simulink model "Problem1"  (R2020b)
settings: Solver=VariableStepAuto  StartTime=0.0  StopTime=10  RelTol=1e-3
model workspace (MAT data in the model file):
  b = 50
  k1 = 50
  k12 = 25
  m1 = 100
  m2 = 4
settings Model: ModifiedByFormat=Dell  Creator=Dell  LastModifiedBy=Dell

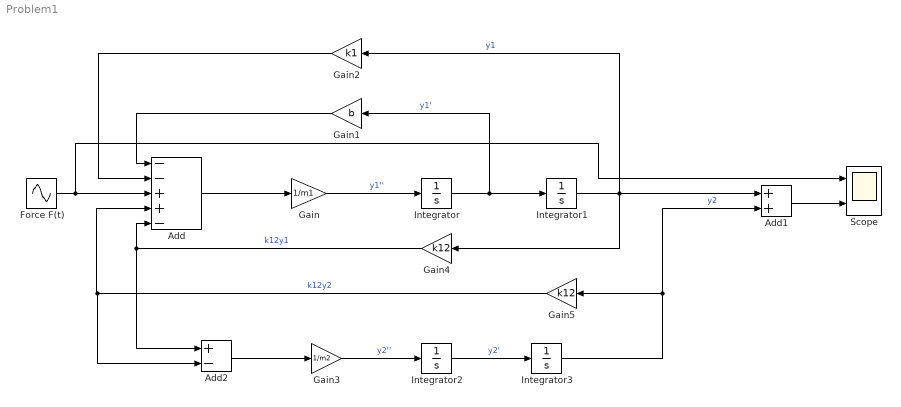
== system Problem1 ==
  Add : Sum  Inputs=--++-
  Add1 : Sum
  Add2 : Sum  Inputs=+-
  Force F(t) : Sin  Amplitude=2  Frequency=10  SampleTime=0
  Gain : Gain  Gain=1/m1
  Gain1 : Gain  Gain=b
  Gain2 : Gain  Gain=k1
  Gain3 : Gain  Gain=1/m2
  Gain4 : Gain  Gain=k12
  Gain5 : Gain  Gain=k12
  Integrator{,1..3} (4 alike) : Integrator
  Scope : Scope  NumInputPorts=2
  wires:
  Add/1 -> Gain/1
  Gain/1 -> Integrator/1  "y1''"
  Integrator/1 -> Gain1/1, Integrator1/1  "y1'"
  Integrator1/1 -> Add1/1, Gain2/1, Gain4/1  "y1"
  Force F(t)/1 -> Scope/1, Add/3
  Gain1/1 -> Add/1
  Gain2/1 -> Add/2
  Add2/1 -> Gain3/1
  Gain3/1 -> Integrator2/1  "y2''"
  Integrator2/1 -> Integrator3/1  "y2'"
  Gain5/1 -> Add2/2, Add/4  "k12y2"
  Integrator3/1 -> Add1/2, Gain5/1  "y2"
  Gain4/1 -> Add2/1, Add/5  "k12y1"
  Add1/1 -> Scope/2
